simulink model "model2bf"  (R2024b)
settings: Solver=ode4  StartTime=0.0  StopTime=10  FixedStep=2e-3  MaxStep=1e-1  RelTol=1e-3
values from neighbouring files (symbols this model uses):
  Aero = struct    [model2_dim.m]    (also in model2_dim_Chikri.m)
  brake = struct    [model2_dim.m]    (also in model2_dim_Chikri.m)
  drivetrain = struct    [model2_dim.m]    (also in model2_dim_Chikri.m)
  g = 9.81    [model2_dim.m]    (also in model2_dim_Chikri.m)
  G29 = struct    [model2_dim.m]    (also in model2_dim_Chikri.m)
  hub_offset = 2.5    [model2_dim.m]    (also in model2_dim_Chikri.m)
  motor = struct    [model2_dim.m]    (also in model2_dim_Chikri.m)
  slope_angle = 0    [model2_dim.m]    (also in model2_dim_Chikri.m)
  suspension = struct    [model2_dim.m]    (also in model2_dim_Chikri.m)
  tyre = struct    [model2_dim.m]    (also in model2_dim_Chikri.m)
  vehicle = struct    [Dimesnsion.m]    (also in model2_dim.m; model2_dim_Chikri.m)
undefined symbols (not defined in the file or in its folder): table, wheel, X, Y, Z
libraries: sm_lib x154, nesl_utility x46, simulink x9, slrealtimeG29lib x1, Contact_Forces_Lib x1
(part 6 of 6)

== matlab function model2bf/Tyre FR/Magic formula subsystem/MATLAB Function ==
  data: u input; theta output; r input
function theta = fcn(u, r)
% function that calculates the slip angle of the tyre without considering
% the steering input given from the driver
% u = speed of the tyre [ux, uy, uz]
% r = rotation sequence of the tyre frame system [anglearound z-axis, anglearound x-axis, anglearound y-axis]
tyre_direction = exp(1i*r(1));
complexV = u(1) + u(2)*1j;
complexSlip = complexV/tyre_direction;
theta = angle(complexSlip);

== matlab function model2bf/Tyre FR/Magic formula subsystem/Magic formula ==
  data: Fz input; SA input; Fy output; Camber input
function Fy = fcn(Fz, SA, Camber)
% Magic formula based on the data extracted from the TTC files

%valuesOfCamber = [0, 2, 4]
if abs(Camber) < 2
    params = [0.198719422442493, 1.649465431297653, 2.373300291953069, 0.233708623192915];
elseif 2 < abs(Camber) && abs(Camber)< 4
    params =[0.198225281942057, 1.660247836348132, 2.603573409360138, 0.381647688805729];
else
    params = [0.208412365438189, 1.632235951563173, 2.790064934147678, 0.398583330098178];
end
Fy = Fz * (params(3) * sin(params(2) * atan(params(1) * SA - params(4) * (params(1) * SA - atan(params(1) * SA)))));

== matlab function model2bf/Tyre FR/Magic formula subsystem/norm ==
  data: u input; y output
function y = fcn(u)
y = norm(u);

== matlab function model2bf/Tyre_RR/Magic formula subsystem/MATLAB Function ==
  data: u input; theta output; r input
function theta = fcn(u, r)
% function that calculates the slip angle of the tyre without considering
% the steering input given from the driver
% u = speed of the tyre [ux, uy, uz]
% r = rotation sequence of the tyre frame system [anglearound z-axis, anglearound x-axis, anglearound y-axis]
tyre_direction = exp(1i*r(1));
complexV = u(1) + u(2)*1j;
complexSlip = complexV/tyre_direction;
theta = angle(complexSlip);

== matlab function model2bf/Tyre_FL/Magic formula subsystem/norm ==
  data: u input; y output
function y = fcn(u)
y = norm(u);

== matlab function model2bf/Driveline/Acceleration calculation/MATLAB Function ==
  data: maxforce input; limitforce input; wheelforce input; y output
function y = fcn(maxforce, limitforce, wheelforce)
    if wheelforce > maxforce 
        y = limitforce;
    else
        y = wheelforce;
    end
end

== matlab function model2bf/Chassis/Aero Forces/MATLAB Function ==
  data: u input; y output
function y = fcn(u)

y = norm(u);

== matlab function model2bf/Tyre_RR/Magic formula subsystem/Magic formula ==
  data: Fz input; SA input; Fy output; Camber input
function Fy = fcn(Fz, SA, Camber)
% Magic formula based on the data extracted from the TTC files

%valuesOfCamber = [0, 2, 4]
if abs(Camber) < 2
    params = [0.198719422442493, 1.649465431297653, 2.373300291953069, 0.233708623192915];
elseif 2 < abs(Camber) && abs(Camber)< 4
    params =[0.198225281942057, 1.660247836348132, 2.603573409360138, 0.381647688805729];
else
    params = [0.208412365438189, 1.632235951563173, 2.790064934147678, 0.398583330098178];
end
Fy = Fz * (params(3) * sin(params(2) * atan(params(1) * SA - params(4) * (params(1) * SA - atan(params(1) * SA)))));

== matlab function model2bf/Tyre_RR/Magic formula subsystem/norm ==
  data: u input; y output
function y = fcn(u)
y = norm(u);
